simulink model "WaterRunner_closed"  (Simulink 8.1)
settings: Solver=ode23s  StartTime=0.0  StopTime=15  RelTol=1e-3
undefined symbols (not defined in the file): Amp, b_water, cw_FL_HL, cw_FR_FL, cw_FR_HR, cw_HR_HL, dTorqueAmp, dTorqueFreq, Filter_Coef, FL_HL_lag, FR_FL_lag, FR_HR_lag, Fratio, freq, g, HR_HL_lag, K_d, K_e, K_i, K_p, k_water, leg_length, Lx, Lxmat, Lz, Lzmat, mass, mass_matrix, omega_0, stepSizePitch, stepSizeRoll, tail_density, tail_length, tail_pad_radius, water_level, X, Y, y_0, Z
libraries: nesl_utility x38, sm_lib x34, WaterRunner_lib_2 x11, dspstat3 x6, dspinverses x1
(part 4 of 4)

== system WaterRunner_closed/Water Contact FR3/Subsystem/water_model/Subsystem4 ==
  r : Inport
  r0 : Inport  Port=2
  Sum1 : Sum  Inputs=-|+
  Switch : Switch
  r00 : Outport
  wires:
  Switch/1 -> r00/1
  Sum1/1 -> Switch/2
  r0/1 -> Switch/3, Sum1/2
  r/1 -> Switch/1, Sum1/1

== system WaterRunner_closed/Water Contact FR3/Subsystem/water_model/damper_force1 ==
  up_b : Inport
  a : Inport  Port=2
  b : Inport  Port=3
  Constant : Constant  Value=R
  Constant1 : Constant  Value=pi/2
  Gain : Gain  Gain=4
  Gain1 : Gain  Gain=1/8
  Gain2 : Gain  Gain=2/3
  Gain3 : Gain  Gain=1/4
  Mux : Mux  Inputs=2
  Product{,1..3,5} (5 alike) : Product  RndMeth=Zero
  Product4 : Product  Inputs=3  RndMeth=Zero
  Sum{,1..3} (4 alike) : Sum  Inputs=++|
  Sum4 : Sum  Inputs=-+|
  cube : Fcn  Expr=u(1)^3
  l(r) : Fcn  Expr=sqrt(u(2)^2-u(1)^2)
  phi(r) : Fcn  Expr=asin(u(1)/u(2))
  sq : Fcn  Expr=u(1)^2
  sq1 : Fcn  Expr=u(1)^2
  sq2 : Fcn  Expr=u(1)^2
  Int_b : Outport
  wires:
  Sum4/1 -> Int_b/1
  Product4/1 -> Sum4/1  "al3(a/4+2b/3)"
  Product3/1 -> Sum4/2
  cube/1 -> Product4/3
  Sum3/1 -> Product4/2
  Gain3/1 -> Sum3/1
  Gain2/1 -> Sum3/2
  Sum2/1 -> Product3/2
  Gain1/1 -> Product3/1
  Product2/1 -> Sum2/2
  Product1/1 -> Sum2/1
  l(r)/1 -> Product2/1, cube/1
  sq2/1 -> Product/2, Product1/1
  Sum1/1 -> Product1/2
  Constant1/1 -> Sum1/2
  phi(r)/1 -> Sum1/1
  Mux/1 -> phi(r)/1, l(r)/1
  up_b/1 -> Product5/2, Product2/2, Mux/1
  Sum/1 -> Gain1/1
  Product/1 -> Sum/2
  Gain/1 -> Sum/1
  sq1/1 -> Gain/1
  sq/1 -> Product/1
  Constant/1 -> sq2/1, Mux/2
  a/1 -> Product5/1, Product4/1, sq/1
  b/1 -> Gain2/1, sq1/1
  Product5/1 -> Gain3/1

== system WaterRunner_closed/Water Contact FR3/Subsystem/water_model/damper_force2 ==
  up_b : Inport
  a : Inport  Port=2
  b : Inport  Port=3
  Constant : Constant  Value=R
  Constant1 : Constant  Value=pi/2
  Gain : Gain  Gain=4
  Gain1 : Gain  Gain=1/8
  Gain2 : Gain  Gain=2/3
  Gain3 : Gain  Gain=1/4
  Mux : Mux  Inputs=2
  Product{,1..3,5} (5 alike) : Product  RndMeth=Zero
  Product4 : Product  Inputs=3  RndMeth=Zero
  Sum{,1..3} (4 alike) : Sum  Inputs=++|
  Sum4 : Sum  Inputs=-+|
  cube : Fcn  Expr=u(1)^3
  l(r) : Fcn  Expr=sqrt(u(2)^2-u(1)^2)
  phi(r) : Fcn  Expr=asin(u(1)/u(2))
  sq : Fcn  Expr=u(1)^2
  sq1 : Fcn  Expr=u(1)^2
  sq2 : Fcn  Expr=u(1)^2
  Int_b : Outport
  wires:
  Product5/1 -> Gain3/1
  b/1 -> sq1/1, Gain2/1
  a/1 -> sq/1, Product4/1, Product5/1
  Constant/1 -> Mux/2, sq2/1
  sq/1 -> Product/1
  sq1/1 -> Gain/1
  Gain/1 -> Sum/1
  Product/1 -> Sum/2
  Sum/1 -> Gain1/1
  up_b/1 -> Mux/1, Product2/2, Product5/2
  Mux/1 -> l(r)/1, phi(r)/1
  phi(r)/1 -> Sum1/1
  Constant1/1 -> Sum1/2
  Sum1/1 -> Product1/2
  sq2/1 -> Product1/1, Product/2
  l(r)/1 -> cube/1, Product2/1
  Product1/1 -> Sum2/1
  Product2/1 -> Sum2/2
  Gain1/1 -> Product3/1
  Sum2/1 -> Product3/2
  Gain2/1 -> Sum3/2
  Gain3/1 -> Sum3/1
  Sum3/1 -> Product4/2
  cube/1 -> Product4/3
  Product3/1 -> Sum4/2
  Product4/1 -> Sum4/1  "al3(a/4+2b/3)"
  Sum4/1 -> Int_b/1

== system WaterRunner_closed/Water Contact FR3/Subsystem/water_model/spring_force ==
  up_b : Inport
  a : Inport  Port=2
  b : Inport  Port=3
  Constant : Constant  Value=R
  Gain : Gain  Gain=-1/3
  Gain1 : Gain  Gain=1/2
  Gain2 : Gain  Gain=pi/4
  Gain3 : Gain  Gain=1/2
  Mux : Mux  Inputs=2
  Product : Product  RndMeth=Zero
  Product1 : Product  Inputs=3  RndMeth=Zero
  Product2 : Product  RndMeth=Zero
  Product3 : Product  RndMeth=Zero
  Sum : Sum  Inputs=|++++|
  cube : Fcn  Expr=u(1)^3
  l(r) : Fcn  Expr=sqrt(u(2)^2-u(1)^2)
  phi(r) : Fcn  Expr=asin(u(1)/u(2))
  sq : Fcn  Expr=u(1)^2
  Int_k : Outport
  wires:
  cube/1 -> Product/2
  b/1 -> Product2/1, Product1/1
  Product3/1 -> Gain3/1
  Gain2/1 -> Sum/3
  Gain/1 -> Sum/2
  Sum/1 -> Int_k/1
  Gain3/1 -> Sum/4
  Gain1/1 -> Sum/1
  phi(r)/1 -> Product3/2
  Product/1 -> Gain/1
  up_b/1 -> Product1/2, Mux/1
  Mux/1 -> phi(r)/1, l(r)/1
  Constant/1 -> Mux/2, sq/1
  Product1/1 -> Gain1/1
  l(r)/1 -> Product1/3, cube/1
  a/1 -> Product/1
  sq/1 -> Product2/2
  Product2/1 -> Product3/1, Gain2/1

== system WaterRunner_closed/Water Contact FR3/Subsystem/water_model1/Subsystem ==
  y_c : Inport
  angle : Inport  Port=2
  Constant : Constant  Value=y_w
  Fcn : Fcn  Expr=sin(u(1))
  Fcn1 : Fcn  Expr=u(1)/u(2)
  Mux : Mux  Inputs=2
  Sum : Sum  Inputs=+-|
  sat : Saturate  UpperLimit=R  LowerLimit=-R
  sat1 : Saturate  UpperLimit=pi  LowerLimit=0
  up_b : Outport
  wires:
  Sum/1 -> Mux/1
  angle/1 -> sat1/1
  Fcn1/1 -> sat/1
  y_c/1 -> Sum/2
  Constant/1 -> Sum/1
  Mux/1 -> Fcn1/1
  Fcn/1 -> Mux/2
  sat/1 -> up_b/1
  sat1/1 -> Fcn/1

== system WaterRunner_closed/Water Contact FR3/Subsystem/water_model1/Subsystem1 ==
  y_c : Inport
  angle : Inport  Port=2
  Constant : Constant  Value=y_w
  Fcn : Fcn  Expr=sin(u(1))
  Gain : Gain  Gain=-2*(-g)
  Gain1 : Gain  Gain=2*(-g)
  Sum : Sum  Inputs=-+|
  a : Outport
  b : Outport  Port=2
  wires:
  angle/1 -> Fcn/1
  y_c/1 -> Sum/1
  Sum/1 -> Gain1/1
  Constant/1 -> Sum/2
  Fcn/1 -> Gain/1
  Gain/1 -> a/1
  Gain1/1 -> b/1

== system WaterRunner_closed/Water Contact FR3/Subsystem/water_model1/Subsystem2 ==
  dtheta : Inport
  v : Inport  Port=2
  r0 : Inport  Port=3
  Constant : Constant  Value=100*eps
  Product : Product  RndMeth=Zero
  Product1 : Product  RndMeth=Zero
  Sign : Signum
  Sign1 : Signum
  Sum2 : Sum  Inputs=|++
  Sum3 : Sum  Inputs=|++
  Sum4 : Sum  Inputs=-+|
  Sum5 : Sum  Inputs=++|
  S+ : Outport
  S- : Outport  Port=2
  wires:
  Product/1 -> Sum2/1
  Product1/1 -> Sum3/1
  Sum5/1 -> Product1/1
  Sign1/1 -> S-/1
  r0/1 -> Sum4/2, Sum5/2
  dtheta/1 -> Product/2, Product1/2
  Sign/1 -> S+/1
  v/1 -> Sum2/2, Sum3/2
  Sum4/1 -> Product/1
  Constant/1 -> Sum4/1, Sum5/1
  Sum3/1 -> Sign/1
  Sum2/1 -> Sign1/1

== system WaterRunner_closed/Water Contact FR3/Subsystem/water_model1/Subsystem3 ==
  vel : Inport
  dtheta : Inport  Port=2
  C : Constant  Value=0
  Fcn : Fcn  Expr=-u(1)/(u(2))
  Mux : Mux  Inputs=2
  Switch : Switch
  sat1 : Saturate  UpperLimit=R  LowerLimit=-R
  mid_b : Outport
  wires:
  C/1 -> Switch/1
  Switch/1 -> sat1/1
  Fcn/1 -> Switch/3
  sat1/1 -> mid_b/1
  vel/1 -> Mux/1
  dtheta/1 -> Mux/2, Switch/2
  Mux/1 -> Fcn/1

== system WaterRunner_closed/Water Contact FR3/Subsystem/water_model1/Subsystem4 ==
  r : Inport
  r0 : Inport  Port=2
  Sum1 : Sum  Inputs=-|+
  Switch : Switch
  r00 : Outport
  wires:
  Switch/1 -> r00/1
  Sum1/1 -> Switch/2
  r0/1 -> Switch/3, Sum1/2
  r/1 -> Switch/1, Sum1/1

== system WaterRunner_closed/Water Contact FR3/Subsystem/water_model1/damper_force1 ==
  up_b : Inport
  a : Inport  Port=2
  b : Inport  Port=3
  Constant : Constant  Value=R
  Constant1 : Constant  Value=pi/2
  Gain : Gain  Gain=4
  Gain1 : Gain  Gain=1/8
  Gain2 : Gain  Gain=2/3
  Gain3 : Gain  Gain=1/4
  Mux : Mux  Inputs=2
  Product{,1..3,5} (5 alike) : Product  RndMeth=Zero
  Product4 : Product  Inputs=3  RndMeth=Zero
  Sum{,1..3} (4 alike) : Sum  Inputs=++|
  Sum4 : Sum  Inputs=-+|
  cube : Fcn  Expr=u(1)^3
  l(r) : Fcn  Expr=sqrt(u(2)^2-u(1)^2)
  phi(r) : Fcn  Expr=asin(u(1)/u(2))
  sq : Fcn  Expr=u(1)^2
  sq1 : Fcn  Expr=u(1)^2
  sq2 : Fcn  Expr=u(1)^2
  Int_b : Outport
  wires:
  Sum4/1 -> Int_b/1
  Product4/1 -> Sum4/1  "al3(a/4+2b/3)"
  Product3/1 -> Sum4/2
  cube/1 -> Product4/3
  Sum3/1 -> Product4/2
  Gain3/1 -> Sum3/1
  Gain2/1 -> Sum3/2
  Sum2/1 -> Product3/2
  Gain1/1 -> Product3/1
  Product2/1 -> Sum2/2
  Product1/1 -> Sum2/1
  l(r)/1 -> Product2/1, cube/1
  sq2/1 -> Product/2, Product1/1
  Sum1/1 -> Product1/2
  Constant1/1 -> Sum1/2
  phi(r)/1 -> Sum1/1
  Mux/1 -> phi(r)/1, l(r)/1
  up_b/1 -> Product5/2, Product2/2, Mux/1
  Sum/1 -> Gain1/1
  Product/1 -> Sum/2
  Gain/1 -> Sum/1
  sq1/1 -> Gain/1
  sq/1 -> Product/1
  Constant/1 -> sq2/1, Mux/2
  a/1 -> Product5/1, Product4/1, sq/1
  b/1 -> Gain2/1, sq1/1
  Product5/1 -> Gain3/1

== system WaterRunner_closed/Water Contact FR3/Subsystem/water_model1/damper_force2 ==
  up_b : Inport
  a : Inport  Port=2
  b : Inport  Port=3
  Constant : Constant  Value=R
  Constant1 : Constant  Value=pi/2
  Gain : Gain  Gain=4
  Gain1 : Gain  Gain=1/8
  Gain2 : Gain  Gain=2/3
  Gain3 : Gain  Gain=1/4
  Mux : Mux  Inputs=2
  Product{,1..3,5} (5 alike) : Product  RndMeth=Zero
  Product4 : Product  Inputs=3  RndMeth=Zero
  Sum{,1..3} (4 alike) : Sum  Inputs=++|
  Sum4 : Sum  Inputs=-+|
  cube : Fcn  Expr=u(1)^3
  l(r) : Fcn  Expr=sqrt(u(2)^2-u(1)^2)
  phi(r) : Fcn  Expr=asin(u(1)/u(2))
  sq : Fcn  Expr=u(1)^2
  sq1 : Fcn  Expr=u(1)^2
  sq2 : Fcn  Expr=u(1)^2
  Int_b : Outport
  wires:
  Product5/1 -> Gain3/1
  b/1 -> sq1/1, Gain2/1
  a/1 -> sq/1, Product4/1, Product5/1
  Constant/1 -> Mux/2, sq2/1
  sq/1 -> Product/1
  sq1/1 -> Gain/1
  Gain/1 -> Sum/1
  Product/1 -> Sum/2
  Sum/1 -> Gain1/1
  up_b/1 -> Mux/1, Product2/2, Product5/2
  Mux/1 -> l(r)/1, phi(r)/1
  phi(r)/1 -> Sum1/1
  Constant1/1 -> Sum1/2
  Sum1/1 -> Product1/2
  sq2/1 -> Product1/1, Product/2
  l(r)/1 -> cube/1, Product2/1
  Product1/1 -> Sum2/1
  Product2/1 -> Sum2/2
  Gain1/1 -> Product3/1
  Sum2/1 -> Product3/2
  Gain2/1 -> Sum3/2
  Gain3/1 -> Sum3/1
  Sum3/1 -> Product4/2
  cube/1 -> Product4/3
  Product3/1 -> Sum4/2
  Product4/1 -> Sum4/1  "al3(a/4+2b/3)"
  Sum4/1 -> Int_b/1

== system WaterRunner_closed/Water Contact FR3/Subsystem/water_model1/spring_force ==
  up_b : Inport
  a : Inport  Port=2
  b : Inport  Port=3
  Constant : Constant  Value=R
  Gain : Gain  Gain=-1/3
  Gain1 : Gain  Gain=1/2
  Gain2 : Gain  Gain=pi/4
  Gain3 : Gain  Gain=1/2
  Mux : Mux  Inputs=2
  Product : Product  RndMeth=Zero
  Product1 : Product  Inputs=3  RndMeth=Zero
  Product2 : Product  RndMeth=Zero
  Product3 : Product  RndMeth=Zero
  Sum : Sum  Inputs=|++++|
  cube : Fcn  Expr=u(1)^3
  l(r) : Fcn  Expr=sqrt(u(2)^2-u(1)^2)
  phi(r) : Fcn  Expr=asin(u(1)/u(2))
  sq : Fcn  Expr=u(1)^2
  Int_k : Outport
  wires:
  cube/1 -> Product/2
  b/1 -> Product2/1, Product1/1
  Product3/1 -> Gain3/1
  Gain2/1 -> Sum/3
  Gain/1 -> Sum/2
  Sum/1 -> Int_k/1
  Gain3/1 -> Sum/4
  Gain1/1 -> Sum/1
  phi(r)/1 -> Product3/2
  Product/1 -> Gain/1
  up_b/1 -> Product1/2, Mux/1
  Mux/1 -> phi(r)/1, l(r)/1
  Constant/1 -> Mux/2, sq/1
  Product1/1 -> Gain1/1
  l(r)/1 -> Product1/3, cube/1
  a/1 -> Product/1
  sq/1 -> Product2/2
  Product2/1 -> Product3/1, Gain2/1

== system WaterRunner_closed/Water Contact FR4/Subsystem/water_model/Subsystem ==
  y_c : Inport
  angle : Inport  Port=2
  Constant : Constant  Value=y_w
  Fcn : Fcn  Expr=sin(u(1))
  Fcn1 : Fcn  Expr=u(1)/u(2)
  Mux : Mux  Inputs=2
  Sum : Sum  Inputs=+-|
  sat : Saturate  UpperLimit=R  LowerLimit=-R
  sat1 : Saturate  UpperLimit=pi  LowerLimit=0
  up_b : Outport
  wires:
  Sum/1 -> Mux/1
  Fcn1/1 -> sat/1
  y_c/1 -> Sum/2
  Constant/1 -> Sum/1
  Mux/1 -> Fcn1/1
  Fcn/1 -> Mux/2
  sat/1 -> up_b/1
  angle/1 -> sat1/1
  sat1/1 -> Fcn/1

== system WaterRunner_closed/Water Contact FR4/Subsystem/water_model/Subsystem1 ==
  y_c : Inport
  angle : Inport  Port=2
  Constant : Constant  Value=y_w
  Fcn : Fcn  Expr=sin(u(1))
  Gain : Gain  Gain=-2*(-g)
  Gain1 : Gain  Gain=2*(-g)
  Sum : Sum  Inputs=-+|
  a : Outport
  b : Outport  Port=2
  wires:
  angle/1 -> Fcn/1
  y_c/1 -> Sum/1
  Sum/1 -> Gain1/1
  Constant/1 -> Sum/2
  Fcn/1 -> Gain/1
  Gain/1 -> a/1
  Gain1/1 -> b/1

== system WaterRunner_closed/Water Contact FR4/Subsystem/water_model/Subsystem2 ==
  dtheta : Inport
  v : Inport  Port=2
  r0 : Inport  Port=3
  Constant : Constant  Value=100*eps
  Product : Product  RndMeth=Zero
  Product1 : Product  RndMeth=Zero
  Sign : Signum
  Sign1 : Signum
  Sum2 : Sum  Inputs=|++
  Sum3 : Sum  Inputs=|++
  Sum4 : Sum  Inputs=-+|
  Sum5 : Sum  Inputs=++|
  S+ : Outport
  S- : Outport  Port=2
  wires:
  Product/1 -> Sum2/1
  Product1/1 -> Sum3/1
  Sum5/1 -> Product1/1
  Sign1/1 -> S-/1
  r0/1 -> Sum4/2, Sum5/2
  dtheta/1 -> Product/2, Product1/2
  Sign/1 -> S+/1
  v/1 -> Sum2/2, Sum3/2
  Sum4/1 -> Product/1
  Constant/1 -> Sum4/1, Sum5/1
  Sum3/1 -> Sign/1
  Sum2/1 -> Sign1/1

== system WaterRunner_closed/Water Contact FR4/Subsystem/water_model/Subsystem3 ==
  vel : Inport
  dtheta : Inport  Port=2
  C : Constant  Value=0
  Fcn : Fcn  Expr=-u(1)/(u(2))
  Mux : Mux  Inputs=2
  Switch : Switch
  sat1 : Saturate  UpperLimit=R  LowerLimit=-R
  mid_b : Outport
  wires:
  C/1 -> Switch/1
  Switch/1 -> sat1/1
  Fcn/1 -> Switch/3
  sat1/1 -> mid_b/1
  vel/1 -> Mux/1
  dtheta/1 -> Mux/2, Switch/2
  Mux/1 -> Fcn/1

== system WaterRunner_closed/Water Contact FR4/Subsystem/water_model/Subsystem4 ==
  r : Inport
  r0 : Inport  Port=2
  Sum1 : Sum  Inputs=-|+
  Switch : Switch
  r00 : Outport
  wires:
  Switch/1 -> r00/1
  Sum1/1 -> Switch/2
  r0/1 -> Switch/3, Sum1/2
  r/1 -> Switch/1, Sum1/1

== system WaterRunner_closed/Water Contact FR4/Subsystem/water_model/damper_force1 ==
  up_b : Inport
  a : Inport  Port=2
  b : Inport  Port=3
  Constant : Constant  Value=R
  Constant1 : Constant  Value=pi/2
  Gain : Gain  Gain=4
  Gain1 : Gain  Gain=1/8
  Gain2 : Gain  Gain=2/3
  Gain3 : Gain  Gain=1/4
  Mux : Mux  Inputs=2
  Product{,1..3,5} (5 alike) : Product  RndMeth=Zero
  Product4 : Product  Inputs=3  RndMeth=Zero
  Sum{,1..3} (4 alike) : Sum  Inputs=++|
  Sum4 : Sum  Inputs=-+|
  cube : Fcn  Expr=u(1)^3
  l(r) : Fcn  Expr=sqrt(u(2)^2-u(1)^2)
  phi(r) : Fcn  Expr=asin(u(1)/u(2))
  sq : Fcn  Expr=u(1)^2
  sq1 : Fcn  Expr=u(1)^2
  sq2 : Fcn  Expr=u(1)^2
  Int_b : Outport
  wires:
  Sum4/1 -> Int_b/1
  Product4/1 -> Sum4/1  "al3(a/4+2b/3)"
  Product3/1 -> Sum4/2
  cube/1 -> Product4/3
  Sum3/1 -> Product4/2
  Gain3/1 -> Sum3/1
  Gain2/1 -> Sum3/2
  Sum2/1 -> Product3/2
  Gain1/1 -> Product3/1
  Product2/1 -> Sum2/2
  Product1/1 -> Sum2/1
  l(r)/1 -> Product2/1, cube/1
  sq2/1 -> Product/2, Product1/1
  Sum1/1 -> Product1/2
  Constant1/1 -> Sum1/2
  phi(r)/1 -> Sum1/1
  Mux/1 -> phi(r)/1, l(r)/1
  up_b/1 -> Product5/2, Product2/2, Mux/1
  Sum/1 -> Gain1/1
  Product/1 -> Sum/2
  Gain/1 -> Sum/1
  sq1/1 -> Gain/1
  sq/1 -> Product/1
  Constant/1 -> sq2/1, Mux/2
  a/1 -> Product5/1, Product4/1, sq/1
  b/1 -> Gain2/1, sq1/1
  Product5/1 -> Gain3/1

== system WaterRunner_closed/Water Contact FR4/Subsystem/water_model/damper_force2 ==
  up_b : Inport
  a : Inport  Port=2
  b : Inport  Port=3
  Constant : Constant  Value=R
  Constant1 : Constant  Value=pi/2
  Gain : Gain  Gain=4
  Gain1 : Gain  Gain=1/8
  Gain2 : Gain  Gain=2/3
  Gain3 : Gain  Gain=1/4
  Mux : Mux  Inputs=2
  Product{,1..3,5} (5 alike) : Product  RndMeth=Zero
  Product4 : Product  Inputs=3  RndMeth=Zero
  Sum{,1..3} (4 alike) : Sum  Inputs=++|
  Sum4 : Sum  Inputs=-+|
  cube : Fcn  Expr=u(1)^3
  l(r) : Fcn  Expr=sqrt(u(2)^2-u(1)^2)
  phi(r) : Fcn  Expr=asin(u(1)/u(2))
  sq : Fcn  Expr=u(1)^2
  sq1 : Fcn  Expr=u(1)^2
  sq2 : Fcn  Expr=u(1)^2
  Int_b : Outport
  wires:
  Product5/1 -> Gain3/1
  b/1 -> sq1/1, Gain2/1
  a/1 -> sq/1, Product4/1, Product5/1
  Constant/1 -> Mux/2, sq2/1
  sq/1 -> Product/1
  sq1/1 -> Gain/1
  Gain/1 -> Sum/1
  Product/1 -> Sum/2
  Sum/1 -> Gain1/1
  up_b/1 -> Mux/1, Product2/2, Product5/2
  Mux/1 -> l(r)/1, phi(r)/1
  phi(r)/1 -> Sum1/1
  Constant1/1 -> Sum1/2
  Sum1/1 -> Product1/2
  sq2/1 -> Product1/1, Product/2
  l(r)/1 -> cube/1, Product2/1
  Product1/1 -> Sum2/1
  Product2/1 -> Sum2/2
  Gain1/1 -> Product3/1
  Sum2/1 -> Product3/2
  Gain2/1 -> Sum3/2
  Gain3/1 -> Sum3/1
  Sum3/1 -> Product4/2
  cube/1 -> Product4/3
  Product3/1 -> Sum4/2
  Product4/1 -> Sum4/1  "al3(a/4+2b/3)"
  Sum4/1 -> Int_b/1

== system WaterRunner_closed/Water Contact FR4/Subsystem/water_model/spring_force ==
  up_b : Inport
  a : Inport  Port=2
  b : Inport  Port=3
  Constant : Constant  Value=R
  Gain : Gain  Gain=-1/3
  Gain1 : Gain  Gain=1/2
  Gain2 : Gain  Gain=pi/4
  Gain3 : Gain  Gain=1/2
  Mux : Mux  Inputs=2
  Product : Product  RndMeth=Zero
  Product1 : Product  Inputs=3  RndMeth=Zero
  Product2 : Product  RndMeth=Zero
  Product3 : Product  RndMeth=Zero
  Sum : Sum  Inputs=|++++|
  cube : Fcn  Expr=u(1)^3
  l(r) : Fcn  Expr=sqrt(u(2)^2-u(1)^2)
  phi(r) : Fcn  Expr=asin(u(1)/u(2))
  sq : Fcn  Expr=u(1)^2
  Int_k : Outport
  wires:
  cube/1 -> Product/2
  b/1 -> Product2/1, Product1/1
  Product3/1 -> Gain3/1
  Gain2/1 -> Sum/3
  Gain/1 -> Sum/2
  Sum/1 -> Int_k/1
  Gain3/1 -> Sum/4
  Gain1/1 -> Sum/1
  phi(r)/1 -> Product3/2
  Product/1 -> Gain/1
  up_b/1 -> Product1/2, Mux/1
  Mux/1 -> phi(r)/1, l(r)/1
  Constant/1 -> Mux/2, sq/1
  Product1/1 -> Gain1/1
  l(r)/1 -> Product1/3, cube/1
  a/1 -> Product/1
  sq/1 -> Product2/2
  Product2/1 -> Product3/1, Gain2/1

== system WaterRunner_closed/Water Contact FR4/Subsystem/water_model1/Subsystem ==
  y_c : Inport
  angle : Inport  Port=2
  Constant : Constant  Value=y_w
  Fcn : Fcn  Expr=sin(u(1))
  Fcn1 : Fcn  Expr=u(1)/u(2)
  Mux : Mux  Inputs=2
  Sum : Sum  Inputs=+-|
  sat : Saturate  UpperLimit=R  LowerLimit=-R
  sat1 : Saturate  UpperLimit=pi  LowerLimit=0
  up_b : Outport
  wires:
  Sum/1 -> Mux/1
  angle/1 -> sat1/1
  Fcn1/1 -> sat/1
  y_c/1 -> Sum/2
  Constant/1 -> Sum/1
  Mux/1 -> Fcn1/1
  Fcn/1 -> Mux/2
  sat/1 -> up_b/1
  sat1/1 -> Fcn/1

== system WaterRunner_closed/Water Contact FR4/Subsystem/water_model1/Subsystem1 ==
  y_c : Inport
  angle : Inport  Port=2
  Constant : Constant  Value=y_w
  Fcn : Fcn  Expr=sin(u(1))
  Gain : Gain  Gain=-2*(-g)
  Gain1 : Gain  Gain=2*(-g)
  Sum : Sum  Inputs=-+|
  a : Outport
  b : Outport  Port=2
  wires:
  angle/1 -> Fcn/1
  y_c/1 -> Sum/1
  Sum/1 -> Gain1/1
  Constant/1 -> Sum/2
  Fcn/1 -> Gain/1
  Gain/1 -> a/1
  Gain1/1 -> b/1

== system WaterRunner_closed/Water Contact FR4/Subsystem/water_model1/Subsystem2 ==
  dtheta : Inport
  v : Inport  Port=2
  r0 : Inport  Port=3
  Constant : Constant  Value=100*eps
  Product : Product  RndMeth=Zero
  Product1 : Product  RndMeth=Zero
  Sign : Signum
  Sign1 : Signum
  Sum2 : Sum  Inputs=|++
  Sum3 : Sum  Inputs=|++
  Sum4 : Sum  Inputs=-+|
  Sum5 : Sum  Inputs=++|
  S+ : Outport
  S- : Outport  Port=2
  wires:
  Product/1 -> Sum2/1
  Product1/1 -> Sum3/1
  Sum5/1 -> Product1/1
  Sign1/1 -> S-/1
  r0/1 -> Sum4/2, Sum5/2
  dtheta/1 -> Product/2, Product1/2
  Sign/1 -> S+/1
  v/1 -> Sum2/2, Sum3/2
  Sum4/1 -> Product/1
  Constant/1 -> Sum4/1, Sum5/1
  Sum3/1 -> Sign/1
  Sum2/1 -> Sign1/1

== system WaterRunner_closed/Water Contact FR4/Subsystem/water_model1/Subsystem3 ==
  vel : Inport
  dtheta : Inport  Port=2
  C : Constant  Value=0
  Fcn : Fcn  Expr=-u(1)/(u(2))
  Mux : Mux  Inputs=2
  Switch : Switch
  sat1 : Saturate  UpperLimit=R  LowerLimit=-R
  mid_b : Outport
  wires:
  C/1 -> Switch/1
  Switch/1 -> sat1/1
  Fcn/1 -> Switch/3
  sat1/1 -> mid_b/1
  vel/1 -> Mux/1
  dtheta/1 -> Mux/2, Switch/2
  Mux/1 -> Fcn/1

== system WaterRunner_closed/Water Contact FR4/Subsystem/water_model1/Subsystem4 ==
  r : Inport
  r0 : Inport  Port=2
  Sum1 : Sum  Inputs=-|+
  Switch : Switch
  r00 : Outport
  wires:
  Switch/1 -> r00/1
  Sum1/1 -> Switch/2
  r0/1 -> Switch/3, Sum1/2
  r/1 -> Switch/1, Sum1/1

== system WaterRunner_closed/Water Contact FR4/Subsystem/water_model1/damper_force1 ==
  up_b : Inport
  a : Inport  Port=2
  b : Inport  Port=3
  Constant : Constant  Value=R
  Constant1 : Constant  Value=pi/2
  Gain : Gain  Gain=4
  Gain1 : Gain  Gain=1/8
  Gain2 : Gain  Gain=2/3
  Gain3 : Gain  Gain=1/4
  Mux : Mux  Inputs=2
  Product{,1..3,5} (5 alike) : Product  RndMeth=Zero
  Product4 : Product  Inputs=3  RndMeth=Zero
  Sum{,1..3} (4 alike) : Sum  Inputs=++|
  Sum4 : Sum  Inputs=-+|
  cube : Fcn  Expr=u(1)^3
  l(r) : Fcn  Expr=sqrt(u(2)^2-u(1)^2)
  phi(r) : Fcn  Expr=asin(u(1)/u(2))
  sq : Fcn  Expr=u(1)^2
  sq1 : Fcn  Expr=u(1)^2
  sq2 : Fcn  Expr=u(1)^2
  Int_b : Outport
  wires:
  Sum4/1 -> Int_b/1
  Product4/1 -> Sum4/1  "al3(a/4+2b/3)"
  Product3/1 -> Sum4/2
  cube/1 -> Product4/3
  Sum3/1 -> Product4/2
  Gain3/1 -> Sum3/1
  Gain2/1 -> Sum3/2
  Sum2/1 -> Product3/2
  Gain1/1 -> Product3/1
  Product2/1 -> Sum2/2
  Product1/1 -> Sum2/1
  l(r)/1 -> Product2/1, cube/1
  sq2/1 -> Product/2, Product1/1
  Sum1/1 -> Product1/2
  Constant1/1 -> Sum1/2
  phi(r)/1 -> Sum1/1
  Mux/1 -> phi(r)/1, l(r)/1
  up_b/1 -> Product5/2, Product2/2, Mux/1
  Sum/1 -> Gain1/1
  Product/1 -> Sum/2
  Gain/1 -> Sum/1
  sq1/1 -> Gain/1
  sq/1 -> Product/1
  Constant/1 -> sq2/1, Mux/2
  a/1 -> Product5/1, Product4/1, sq/1
  b/1 -> Gain2/1, sq1/1
  Product5/1 -> Gain3/1

== system WaterRunner_closed/Water Contact FR4/Subsystem/water_model1/damper_force2 ==
  up_b : Inport
  a : Inport  Port=2
  b : Inport  Port=3
  Constant : Constant  Value=R
  Constant1 : Constant  Value=pi/2
  Gain : Gain  Gain=4
  Gain1 : Gain  Gain=1/8
  Gain2 : Gain  Gain=2/3
  Gain3 : Gain  Gain=1/4
  Mux : Mux  Inputs=2
  Product{,1..3,5} (5 alike) : Product  RndMeth=Zero
  Product4 : Product  Inputs=3  RndMeth=Zero
  Sum{,1..3} (4 alike) : Sum  Inputs=++|
  Sum4 : Sum  Inputs=-+|
  cube : Fcn  Expr=u(1)^3
  l(r) : Fcn  Expr=sqrt(u(2)^2-u(1)^2)
  phi(r) : Fcn  Expr=asin(u(1)/u(2))
  sq : Fcn  Expr=u(1)^2
  sq1 : Fcn  Expr=u(1)^2
  sq2 : Fcn  Expr=u(1)^2
  Int_b : Outport
  wires:
  Product5/1 -> Gain3/1
  b/1 -> sq1/1, Gain2/1
  a/1 -> sq/1, Product4/1, Product5/1
  Constant/1 -> Mux/2, sq2/1
  sq/1 -> Product/1
  sq1/1 -> Gain/1
  Gain/1 -> Sum/1
  Product/1 -> Sum/2
  Sum/1 -> Gain1/1
  up_b/1 -> Mux/1, Product2/2, Product5/2
  Mux/1 -> l(r)/1, phi(r)/1
  phi(r)/1 -> Sum1/1
  Constant1/1 -> Sum1/2
  Sum1/1 -> Product1/2
  sq2/1 -> Product1/1, Product/2
  l(r)/1 -> cube/1, Product2/1
  Product1/1 -> Sum2/1
  Product2/1 -> Sum2/2
  Gain1/1 -> Product3/1
  Sum2/1 -> Product3/2
  Gain2/1 -> Sum3/2
  Gain3/1 -> Sum3/1
  Sum3/1 -> Product4/2
  cube/1 -> Product4/3
  Product3/1 -> Sum4/2
  Product4/1 -> Sum4/1  "al3(a/4+2b/3)"
  Sum4/1 -> Int_b/1

== system WaterRunner_closed/Water Contact FR4/Subsystem/water_model1/spring_force ==
  up_b : Inport
  a : Inport  Port=2
  b : Inport  Port=3
  Constant : Constant  Value=R
  Gain : Gain  Gain=-1/3
  Gain1 : Gain  Gain=1/2
  Gain2 : Gain  Gain=pi/4
  Gain3 : Gain  Gain=1/2
  Mux : Mux  Inputs=2
  Product : Product  RndMeth=Zero
  Product1 : Product  Inputs=3  RndMeth=Zero
  Product2 : Product  RndMeth=Zero
  Product3 : Product  RndMeth=Zero
  Sum : Sum  Inputs=|++++|
  cube : Fcn  Expr=u(1)^3
  l(r) : Fcn  Expr=sqrt(u(2)^2-u(1)^2)
  phi(r) : Fcn  Expr=asin(u(1)/u(2))
  sq : Fcn  Expr=u(1)^2
  Int_k : Outport
  wires:
  cube/1 -> Product/2
  b/1 -> Product2/1, Product1/1
  Product3/1 -> Gain3/1
  Gain2/1 -> Sum/3
  Gain/1 -> Sum/2
  Sum/1 -> Int_k/1
  Gain3/1 -> Sum/4
  Gain1/1 -> Sum/1
  phi(r)/1 -> Product3/2
  Product/1 -> Gain/1
  up_b/1 -> Product1/2, Mux/1
  Mux/1 -> phi(r)/1, l(r)/1
  Constant/1 -> Mux/2, sq/1
  Product1/1 -> Gain1/1
  l(r)/1 -> Product1/3, cube/1
  a/1 -> Product/1
  sq/1 -> Product2/2
  Product2/1 -> Product3/1, Gain2/1
